simulink model "eCS_Algo_Simulation"  (R2018a)
settings: Solver=ode1  StartTime=0.0  StopTime=0.2  FixedStep=1/80000  RelTol=1e-3  EnableMultiTasking=on
PostLoadFcn:
  | , if any(exist('dsrtsu_mdlpostloadfcn', 'file') == [2, 3, 6]), try dsrtsu_mdlpostloadfcn('Execute', bdroot); catch fprintf('Error in PostLoadFcn (dsrtsu_mdlpostloadfcn) for model "%s":\n %s\n', bdroot, lasterr); end, end,
values from neighbouring files (symbols this model uses):
  AccSensor = 5    [Parameter_eCS_Algo.m]
  AlgoType = 0    [Parameter_eCS_Algo.m]
  Cxy = 1*0.017    (= 0.017)    [Acc_Init_SelV1.m]
  Cxz = 1*0.017    (= 0.017)    [Acc_Init_SelV1.m]
  Cyx = 1*0.017    (= 0.017)    [Acc_Init_SelV1.m]
  Cyz = 1*0.017    (= 0.017)    [Acc_Init_SelV1.m]
  Czx = 1*0.017    (= 0.017)    [Acc_Init_SelV1.m]
  Czy = 1*0.017    (= 0.017)    [Acc_Init_SelV1.m]
  FreqTemperature = 10    [Acc_Init_SelV1.m]
  MaxSensorOffset = 0.3    [Acc_Init_SelV1.m]
  Mean_x_noise = 4e-3    (= 0.004)    [Acc_Init_SelV1.m]
  Mean_y_noise = 4e-3    (= 0.004)    [Acc_Init_SelV1.m]
  Mean_z_noise = 4e-3    (= 0.004)    [Acc_Init_SelV1.m]
  ODR = 8000    [Acc_Init_SelV1.m]
  offsetcorrection_on_off = 0    [Parameter_eCS_Algo.m]
  pulsetype = 2    [Parameter_eCS_Algo.m]    (also in run_simulation.m = j; run_simulation_ActiveX.m = j)
  Range = 4    [Acc_Init_SelV1.m]
  TempBias = 0    [Acc_Init_SelV1.m]
  TemperatureAmp = 0    [Acc_Init_SelV1.m]
  Var_x_noise = 1.84e-9    (= 1.84e-09)    [Acc_Init_SelV1.m]
  Var_y_noise = 2.025e-09    [Acc_Init_SelV1.m]
  Var_z_noise = 1.374e-09    [Acc_Init_SelV1.m]
  w_x = 2*pi*F_x    (= 376.991118431)    [Acc_Init_SelV1.m]
  w_y = 2*pi*F_y    (= 376.991118431)    [Acc_Init_SelV1.m]
  w_z = 2*pi*F_z    (= 376.991118431)    [Acc_Init_SelV1.m]
  x_max_temp_drift = 0.061    [Acc_Init_SelV1.m]
  x_offset_enable = 0    [Acc_Init_SelV1.m]
  x_run_to_run_drift = 0.0    (= 0)    [Acc_Init_SelV1.m]
  x_temp_co_drift = 0.000    (= 0)    [Acc_Init_SelV1.m]
  Xi_x = 0.7    [Acc_Init_SelV1.m]
  Xi_y = 0.7    [Acc_Init_SelV1.m]
  Xi_z = 0.7    [Acc_Init_SelV1.m]
  y_max_temp_drift = 0.061    [Acc_Init_SelV1.m]
  y_offset_enable = 0    [Acc_Init_SelV1.m]
  y_run_to_run_drift = 0.0    (= 0)    [Acc_Init_SelV1.m]
  y_temp_co_drift = 0.000    (= 0)    [Acc_Init_SelV1.m]
  z_max_temp_drift = 0.13    [Acc_Init_SelV1.m]
  z_offset_enable = 0    [Acc_Init_SelV1.m]
  z_run_to_run_drift = 0.0    (= 0)    [Acc_Init_SelV1.m]
  z_temp_co_drift = 0.000    (= 0)    [Acc_Init_SelV1.m]
undefined symbols (not defined in the file or in its folder): controller_sample_rate, DiscIntNeverNeededParam, gmw_roada_x__m_s__, gmw_roada_y__m_s__, gmw_roadtime_2kHz, Meldorf_HindenburgstraAcceleration_x__m_s_2_, Meldorf_HindenburgstraAcceleration_y__m_s_2_, Meldorf_HindenburgstraTime__s_, pulse_FF27, pulse_MPDB, pulse_ODB40, pulse_ODB64, pulse_USNCAP, pulsetime_FF27, pulsetime_MPDB, pulsetime_ODB40, pulsetime_ODB64, pulsetime_USNCAP, sigbuilder_block, VW_416_2kHza_x_2kHz, VW_416_2kHza_y_2kHz, VW_416_2kHztime_2kHz
libraries: simulink x23, dspsigops x1
(part 1 of 2)
settings Model: DSRTSU_INTERNAL_RTI_VER=520  DSRTSU_INTERNAL_RTI_TYPE=rti1103  DSRTSU_INTERNAL_RTIFPGA=110  RTICANMMDATA=struct('GeneralSetupData',struct('modelroot','P:\ES\USER\Hinrichs\Projekte\93D48_eCS\Simulink','generalsettings',struct('filesettings',struct('destfolder',struct('Name','RTICANMM_FILES','Check',1),'buildfolder',struct('Name','.','Check',1),'AbsDestfolder',struct('Name','P:\ES\USER\Hinrichs\Projekte\93D48_eCS\Simulink\RTICANMM_FILES'),'AbsBuildfolder',struct('Name','P:\ES\USER\Hinrichs\Projekte\93D48_eCS\Simulink'))),'options',struct('addpaths',1,'rmpaths',1,'addtrcexclusion',logical(1),'cannavigator',struct('checkmonitoring',0),'show_usrtrc',0,'use_usrtrc',0),'advanced',struct('options',[1 1 1 1 1 1 1 1 1 1 1 1 1 1 1 1 1 1 1 1 1 1 1 1 1 1 1 1 1 1 1 1 1 1 1 1 1 1 1 1 1 1 1 1 1 1 1 1 1 1 1 1 1 1 1 1 1 1 1 1 1 1 1 1 1 1 1 1 1 1 1 1 1 1 1 1 1 1 1 1 1 1 1 1 1 1 1 1 1 1 1 1 1 1 1 1 1 1 1 1]),'MPSetup',{{}},'modelname','eCS_Algo_Simulation','block','eCS_Algo_Simulation'))  DSRTSU_INTERNAL_RTIFLEXRAYCONFIG=110  Creator=heiko.hinrichs  LastModifiedBy=Heiko.Hinrichs
settings SolverCC: AutoInsertRateTranBlk=on
settings DataIOCC: LimitDataPoints=on  SaveFormat=Array  SignalLoggingSaveFormat=ModelDataLogs
settings OptimizationCC: BlockReduction=off  OptimizeBlockIOStorage=off  BufferReuse=off  GlobalBufferReuse=off  ExpressionFolding=off  ExpressionDepthLimit=2147483647  LocalBlockOutputs=off  LifeSpan=inf  OptimizeDataStoreBuffers=off  BusAssignmentInplaceUpdate=off
settings DebuggingCC: UnderspecifiedInitializationDetection=Classic  MergeDetectMultiDrivingBlocksExec=none  SolverPrmCheckMsg=warning  FcnCallInpInsideContextMsg=warning  StateNameClashWarn=warning  SFUnexpectedBacktrackingDiag=warning  SFNoUnconditionalDefaultTransitionDiag=warning  SFExecutionAtInitializationDiag=none
settings HardwareCC: ProdBitPerPointer=32  ProdBitPerSizeT=32  ProdBitPerPtrDiffT=32  ProdLargestAtomicInteger=Integer  ProdEndianess=BigEndian  ProdWordSize=32  ProdHWDeviceType=Custom Processor->Custom  TargetHWDeviceType=Custom Processor->Custom
settings ModelReferenceCC: PropagateSignalLabelsOutOfModel=off
settings SFSimCC: MATLABDynamicMemAlloc=off
settings RTWCC: SystemTargetFile=rti1103.tlc  MakeCommand=make_rti  TemplateMakefile=rti1103.tmf  Description=dSPACE DS1103 Hardware Platform
settings CodeAppCC: StateflowObjectComments=on
settings STFCustomTargetCC: ParMdlRefBuildCompliant=on  GRTInterface=off  SystemTargetFile=rti1103.tlc
settings GRTTargetCC: TargetLangStandard=C89/C90 (ANSI)  CompOptLevelCompliant=off  ConcurrentExecutionCompliant=off  CombineOutputUpdateFcns=off  MatFileLogging=off  CPPClassGenCompliant=off  UseToolchainInfoCompliant=off  ExtModeMexFile=noextcomm
settings ConfigComp: CovMetricSettings=dw  CovHtmlReporting=on  CovSaveCumulativeToWorkspaceVar=on  CovSaveSingleToWorkspaceVar=on  CovExternalEMLEnable=off

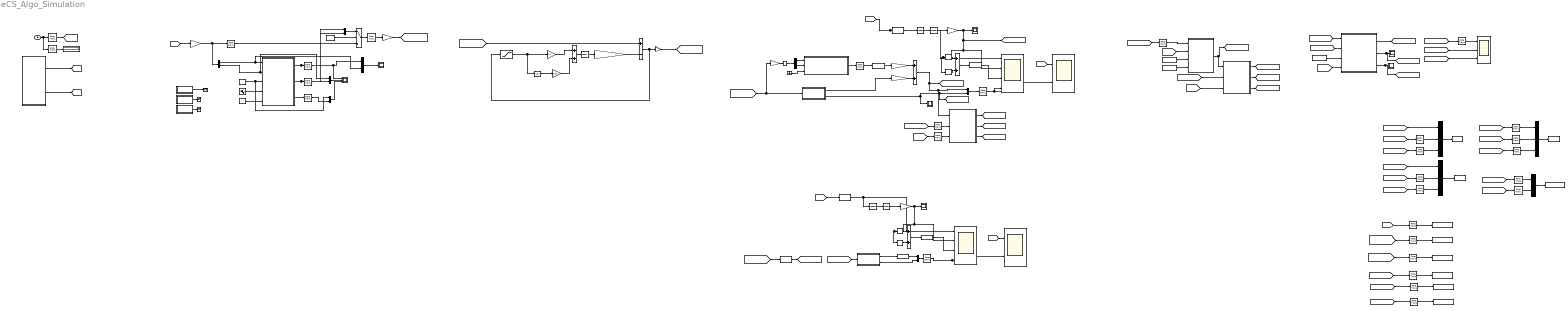
== system eCS_Algo_Simulation ==
  note: "retractor locked"
  note: Outputs
  note: Retractor mechanics
  note: Solenoid
  note: eCS algo
  note: Offset correction
  note: Input pulses / load cases
  note: "old" algo unidirectional
  note: Sensor model Ziad
  note: "lever locked" (solenoid locked)
  note: "lock decision" (algo "locked")
  Accelerometer : Subsystem
  Add{,1,3..4} (4 alike) : Sum
  Add2 : Sum  Inputs=+-
  Clock : Clock
  Compare To Constant : simulink/Logic and Bit Operations/Compare To Constant  relop=>=  const=25  OutDataTypeStr=uint8
  Compare To Constant1 : simulink/Logic and Bit Operations/Compare To Constant  relop=>=  const=50  OutDataTypeStr=uint8
  Compare To Constant2 : simulink/Logic and Bit Operations/Compare To Constant  relop=>=  const=25  OutDataTypeStr=uint8
  Compare To Constant3 : simulink/Logic and Bit Operations/Compare To Constant  relop=>=  const=50  OutDataTypeStr=uint8
  Constant : Constant  Value=0
  Crash signal1 : Subsystem  Tag=STV Subsys  LoadFcn=sigbuilder_block('load');  StartFcn=sigbuilder_block('start');  StopFcn=sigbuilder_block('stop');  ClipboardFcn=sigbuilder_block('clipboard');  mask(Sigbuilder block){tuvar=[0:10]}
      mask help: Simulink:masks:SigbuilderBlock_MD
      mask init:
      | if ~strcmp(get_param(bdroot(gcbh),'SimulationStatus'),'stopped') tuvar = sigbuilder_block('maskInit'); end
      settings: CopyFcn=sigbuilder_block('copy');  DeleteFcn=sigbuilder_block('delete');  ModelCloseFcn=sigbuilder_block('modelClose');  PreSaveFcn=sigbuilder_block('preSave');  PauseFcn=sigbuilder_block('pause');  ContinueFcn=sigbuilder_block('continue');  NameChangeFcn=sigbuilder_block('namechange');  OpenFcn=sigbuilder_block('open',[50.25 1.5 1200 576 ]);  CloseFcn=sigbuilder_block('close');
      mask Display: plot(0, 0, 100, 100,[2, 2, 32, 32, 2], [68, 8, 8, 68, 68],[32, 2], [38, 38], [32, 19, 2],[53, 60, 44], [32, 17, 17, 2],[16, 16, 31, 31]);txt = getActiveGroup(gcbh);text(2, 100, txt,'verticalAlignment', 'top');
  Crash signal3 : Subsystem  Tag=STV Subsys  LoadFcn=sigbuilder_block('load');  StartFcn=sigbuilder_block('start');  StopFcn=sigbuilder_block('stop');  ClipboardFcn=sigbuilder_block('clipboard');  mask(Sigbuilder block){tuvar=[0:10]}
      mask help: Simulink:masks:SigbuilderBlock_MD
      mask init:
      | if ~strcmp(get_param(bdroot(gcbh),'SimulationStatus'),'stopped') tuvar = sigbuilder_block('maskInit'); end
      settings: CopyFcn=sigbuilder_block('copy');  DeleteFcn=sigbuilder_block('delete');  ModelCloseFcn=sigbuilder_block('modelClose');  PreSaveFcn=sigbuilder_block('preSave');  PauseFcn=sigbuilder_block('pause');  ContinueFcn=sigbuilder_block('continue');  NameChangeFcn=sigbuilder_block('namechange');  OpenFcn=sigbuilder_block('open',[54 1.5 1200 540 ]);  CloseFcn=sigbuilder_block('close');
      mask Display: plot(0, 0, 100, 100,[2, 2, 32, 32, 2], [68, 8, 8, 68, 68],[32, 2], [38, 38], [32, 19, 2],[53, 60, 44], [32, 17, 17, 2],[16, 16, 31, 31]);txt = getActiveGroup(gcbh);text(2, 100, txt,'verticalAlignment', 'top');
  Demux : Demux  Outputs=2
  Demux2 : Demux  Outputs=2
  Discrete-Time Integrator{,1..3} (4 alike) : DiscreteIntegrator  SampleTime=-1  ICPrevOutput=DiscIntNeverNeededParam  ICPrevScaledInput=DiscIntNeverNeededParam
  Discrete-Time Integrator4 : DiscreteIntegrator  gainval=1  SampleTime=-1  LimitOutput=on  UpperSaturationLimit=0.3 * 9.81  LowerSaturationLimit=-0.3 * 9.81  ICPrevOutput=DiscIntNeverNeededParam  ICPrevScaledInput=DiscIntNeverNeededParam
  G-lock Scope : Scope  NumInputPorts=4
  G-lock Scope new : Scope  NumInputPorts=4
  Gain : Gain  Gain=AlgoType
  Gain1 : Gain  Gain=1- AlgoType
  Ground : Ground
  Input (Pulse/ Angle) : Subsystem
  Mux : Mux  Inputs=3
  Mux{1,3,5..9} (7 alike) : Mux  Inputs=2
  Mux2 : Mux  Inputs=3
  Mux4 : Mux  Inputs=3
  Noisy : Subsystem  Tag=STV Subsys  LoadFcn=sigbuilder_block('load');  StartFcn=sigbuilder_block('start');  StopFcn=sigbuilder_block('stop');  ClipboardFcn=sigbuilder_block('clipboard');  mask(Sigbuilder block){tuvar=[0:10]}
      mask help: Simulink:masks:SigbuilderBlock_MD
      mask init:
      | if ~strcmp(get_param(bdroot(gcbh),'SimulationStatus'),'stopped') tuvar = sigbuilder_block('maskInit'); end
      settings: CopyFcn=sigbuilder_block('copy');  DeleteFcn=sigbuilder_block('delete');  ModelCloseFcn=sigbuilder_block('modelClose');  PreSaveFcn=sigbuilder_block('preSave');  PauseFcn=sigbuilder_block('pause');  ContinueFcn=sigbuilder_block('continue');  NameChangeFcn=sigbuilder_block('namechange');  OpenFcn=sigbuilder_block('open',[54 1.5 1200 535.5 ]);  CloseFcn=sigbuilder_block('close');
      mask Display: plot(0, 0, 100, 100,[2, 2, 32, 32, 2], [68, 8, 8, 68, 68],[32, 2], [38, 38], [32, 19, 2],[53, 60, 44], [32, 17, 17, 2],[16, 16, 31, 31]);txt = getActiveGroup(gcbh);text(2, 100, txt,'verticalAlignment', 'top');
  Output Scope : Scope  NumInputPorts=3
  Pulse measured : RateTransition
  Pulse measured1 : RateTransition  Deterministic=off  OutPortSampleTime=1/2000
  Pulse measured2 : RateTransition
  Pulse raw (g) : Gain  Gain=1/9.807
  Pulse raw / measured by sensor : Scope
  Pulse raw1 : Gain  Gain=9.807
  Pulse with Offsetcorr. : Gain
  RT : RateTransition  OutPortSampleTime=0.0001
  Rate Transition{,1..11,15,22} (14 alike) : RateTransition
  Rate Transition{12..14,16..21,23..24} (11 alike) : RateTransition  OutPortSampleTime=1/10000
  Rate Transition25 : RateTransition  OutPortSampleTime=1/5
  "Saturation acc. script, i.e.+-0,3g (max. offset of sensor after ageing)" : Saturate  UpperLimit=MaxSensorOffset * 9.807  LowerLimit=-MaxSensorOffset * 9.807
  Scope : Scope
  Scope1 : Scope  NumInputPorts=3
  Sign : Signum
  Temperature : Sin  Amplitude=TemperatureAmp  Bias=TempBias  Frequency=FreqTemperature  SampleTime=0
  Terminator : Terminator
  Terminator2 : Terminator
  Terminator3 : Terminator
  Tilt_Lock_Scop : Scope  NumInputPorts=2
  Tilt_Lock_Scop1 : Scope  NumInputPorts=2
  To Workspace : ToWorkspace  VariableName=triggers_s  SaveFormat=Timeseries  SampleTime=-1
      settings: MaxDataPoints=1  Save2DSignal=2-D array (concatenate along first dimension)
  To Workspace1 : ToWorkspace  VariableName=pulse  SaveFormat=Timeseries  SampleTime=-1
      settings: Save2DSignal=2-D array (concatenate along first dimension)
  To Workspace2 : ToWorkspace  VariableName=pulse_sensor_output  SaveFormat=Timeseries  SampleTime=-1
      settings: Save2DSignal=2-D array (concatenate along first dimension)
  To Workspace3 : ToWorkspace  VariableName=pulse_with_offsetcorrection  SaveFormat=Timeseries  SampleTime=-1
      settings: Save2DSignal=2-D array (concatenate along first dimension)
  To Workspace4 : ToWorkspace  VariableName=s_ball  SaveFormat=Timeseries  SampleTime=-1
      settings: Save2DSignal=2-D array (concatenate along first dimension)
  To Workspace5 : ToWorkspace  VariableName=trigger_eCS  SaveFormat=Timeseries  SampleTime=-1
      settings: Save2DSignal=2-D array (concatenate along first dimension)
  To Workspace6 : ToWorkspace  VariableName=triggers_times  SaveFormat=Timeseries  SampleTime=-1
      settings: MaxDataPoints=1  Save2DSignal=2-D array (concatenate along first dimension)
  To Workspace7 : ToWorkspace  VariableName=s_rig  SaveFormat=Timeseries  SampleTime=-1
      settings: Save2DSignal=2-D array (concatenate along first dimension)
  To Workspace8 : ToWorkspace  VariableName=s_locking  SaveFormat=Timeseries  SampleTime=-1
      settings: Save2DSignal=2-D array (concatenate along first dimension)
  To Workspace9 : ToWorkspace  VariableName=triggercounts  SaveFormat=Timeseries  SampleTime=-1
      settings: Save2DSignal=2-D array (concatenate along first dimension)
  Vektor_addition_Pulse : Fcn  Expr=sqrt( (u(1)*u(1)) + (u(2)*u(2)) )
  Vektor_addition_Pulse1 : Fcn  Expr=sqrt( (u(1)*u(1)) + (u(2)*u(2)) )
  Vektor_addition_Pulse2 : Fcn  Expr=sqrt( (u(1)*u(1)) + (u(2)*u(2)) )
  acc. measurement direct/via acc. sensor : Switch  Criteria=u2 > Threshold
  "acc. sensor type: 0=direct, 1=AD, 2=ST, 3=TDK, 4=NXP" : Constant  Value=AccSensor  VectorParams1D=off
  delta-t to lock (ms) : Constant  Value=5
  delta-t to unlock (ms) : Constant  Value=7
  deviation dependent correction: 0.1/s ~10mg/s at 1m/s²deviation ~0,6°/s with saturation +-0,3g: max. 30mg/s / ~1,8°/s possible : Gain  Gain=0.1
  eCS Algo : Subsystem
  eCS Algo new : Subsystem
  locking distance (mm) : Constant  Value=18.13
  m/s² to g : Gain  Gain=1/9.807
  offset correction on/off : Gain  Gain=offsetcorrection_on_off  OutMin=[0]  OutMax=[1]
  permanent correction: 0.01m/s²/s ~1mg/s ~0,06°/s : Gain  Gain=0.01
  retractor locking trigger : MATLAB Function  TreatAsAtomicUnit=on
  s-locking retractor (mm) : Scope
  s-rig (mm) : Scope
  s-rig (mm) new : Scope
  s-rig-trigger : DataTypeConversion
  s-rig-trigger new : DataTypeConversion
  s-rig-trigger new1 : DataTypeConversion
  s_rig in mm : Gain  Gain=1000
  s_rig in mm1 : Gain  Gain=1000
  solenoid time delay : MATLAB Function  TreatAsAtomicUnit=on
  time (0.2s-steps) : Display
  "trigger travels, times and counts" : MATLAB Function  TreatAsAtomicUnit=on
  "trigger travels, times and counts1" : MATLAB Function  TreatAsAtomicUnit=on
  trigger_lock : DataTypeConversion
  triggertime_retractor (ms) : Scope
  zero 1 : Constant  Value=0
  µC Signalverarbeitung und Algorithmus2 : Subsystem
  wires:
  Mux1/1 -> Rate Transition3/1
  eCS Algo/1(Trigger eCS) -> trigger_lock/1
  Discrete-Time Integrator1/1 -> s_rig in mm/1
  Input (Pulse/ Angle)/1("Pulse_profile ") -> [Pulse]  "pulse in m/s²"
  Discrete-Time Integrator/1 -> Discrete-Time Integrator1/1
  eCS Algo new/2(s_ball) -> [s_ball], Mux3/2, Scope/1
  Add4/1 -> "trigger travels, times and counts"/1(trigger), Mux3/1, [trigger_eCS]
  trigger_lock/1 -> Mux1/1
  eCS Algo/2(s_ball) -> Mux1/2
  s_rig in mm/1 -> [s], G-lock Scope new/2, Compare To Constant/1, Compare To Constant1/1, s-rig (mm) new/1
  [angle] -> Tilt_Lock_Scop/1
  Input (Pulse/ Angle)/2(angle in °) -> [angle]
  Vektor_addition_Pulse/1 -> [Pulse_unidirectional]
  [Pulse_unidirectional] -> eCS Algo/1(Pulse)
  Discrete-Time Integrator2/1 -> Discrete-Time Integrator3/1
  Discrete-Time Integrator3/1 -> s_rig in mm1/1
  Vektor_addition_Pulse2/1 -> Discrete-Time Integrator2/1, G-lock Scope/1
  Compare To Constant/1 -> Add/2
  Compare To Constant1/1 -> Add/1
  Compare To Constant2/1 -> Add1/2
  Compare To Constant3/1 -> Add1/1
  s_rig in mm1/1 -> G-lock Scope/2, Compare To Constant2/1, Compare To Constant3/1, s-rig (mm)/1
  Add1/1 -> s-rig-trigger/1
  s-rig-trigger/1 -> G-lock Scope/3
  Add/1 -> s-rig-trigger new/1
  Mux3/1 -> Rate Transition4/1
  s-rig-trigger new/1 -> G-lock Scope new/3
  "Saturation acc. script, i.e.+-0,3g (max. offset of sensor after ageing)"/1 -> Sign/1, deviation dependent correction: 0.1/s ~10mg/s at 1m/s²deviation ~0,6°/s with saturation +-0,3g: max. 30mg/s / ~1,8°/s possible/1
  Sign/1 -> permanent correction: 0.01m/s²/s ~1mg/s ~0,06°/s/1
  offset correction on/off/1 -> Add2/2
  Discrete-Time Integrator4/1 -> offset correction on/off/1
  Add3/1 -> Discrete-Time Integrator4/1
  deviation dependent correction: 0.1/s ~10mg/s at 1m/s²deviation ~0,6°/s with saturation +-0,3g: max. 30mg/s / ~1,8°/s possible/1 -> Add3/1
  permanent correction: 0.01m/s²/s ~1mg/s ~0,06°/s/1 -> Add3/2
  Add2/1 -> Pulse with Offsetcorr./1, "Saturation acc. script, i.e.+-0,3g (max. offset of sensor after ageing)"/1
  [angle] -> Tilt_Lock_Scop1/1
  Clock/1 -> Rate Transition25/1, Rate Transition2/1
  [time] -> solenoid time delay/2(time)
  [trigger_eCS] -> Rate Transition/1
  solenoid time delay/1(trigger_out) -> "trigger travels, times and counts1"/1(trigger), [locking_solenoid]
  [locking_solenoid] -> Scope1/2
  [trigger_eCS] -> Rate Transition1/1
  Temperature/1 -> Accelerometer/4(Temperature)
  Pulse measured/1 -> Output Scope/1, Mux5/1
  Rate Transition7/1 -> Mux6/2
  Constant/1 -> Accelerometer/5(Max temp. drift)
  Accelerometer/2(Out Y) -> Mux8/2, Rate Transition7/1
  Accelerometer/1(Out X) -> Mux8/1, Pulse measured/1
  Mux7/1 -> Output Scope/3
  Demux2/2 -> Accelerometer/2(In Y), Mux6/1
  Accelerometer/3(Out Z) -> Rate Transition8/1
  zero 1/1 -> Accelerometer/3(In Z), Mux7/1
  Mux6/1 -> Output Scope/2
  Mux5/1 -> Pulse raw / measured by sensor/1
  Crash signal1/1(Signal 1) -> Terminator/1
  Demux2/1 -> Mux5/2, Accelerometer/1(In X)
  Rate Transition8/1 -> Mux7/2
  Pulse with Offsetcorr./1 -> [Pulse_with_offsetcorrection]
  locking distance (mm)/1 -> retractor locking trigger/3(s_mech_locking)
  [time] -> retractor locking trigger/4(time)
  [s] -> retractor locking trigger/2(s)
  [locking_solenoid] -> retractor locking trigger/1(trigger_solenoid)
  [locking_retractor] -> Scope1/3
  retractor locking trigger/1(trigger_retractor) -> [locking_retractor]
  retractor locking trigger/2(triggertime_retractor) -> [triggertime_retractor], triggertime_retractor (ms)/1
  retractor locking trigger/3(s_locking) -> [s_locking_retractor], s-locking retractor (mm)/1
  Pulse measured1/1 -> Pulse raw1/1
  Pulse raw1/1 -> [Pulse_no_offsetcorrection]
  [Pulse_with_offsetcorrection] -> Vektor_addition_Pulse/1
  [Pulse] -> Vektor_addition_Pulse1/1, G-lock Scope new/1
  [Pulse] -> Vektor_addition_Pulse2/1
  Vektor_addition_Pulse1/1 -> Discrete-Time Integrator/1
  [Pulse_no_offsetcorrection] -> Add2/1
  Noisy/1(Signal 1) -> Terminator2/1
  Crash signal3/1(Signal 1) -> Terminator3/1
  Rate Transition/1 -> solenoid time delay/1(trigger)
  Rate Transition1/1 -> Scope1/1
  Mux/1 -> To Workspace/1
  Pulse raw (g)/1 -> Pulse measured2/1, Demux2/1
  Rate Transition2/1 -> [time]
  [Pulse] -> Pulse raw (g)/1
  Rate Transition3/1 -> G-lock Scope/4, Tilt_Lock_Scop/2
  Rate Transition4/1 -> G-lock Scope new/4, Tilt_Lock_Scop1/2
  [time] -> Rate Transition5/1
  Rate Transition5/1 -> "trigger travels, times and counts"/3(time)
  "trigger travels, times and counts"/2(triggertime) -> [triggertime_eCS]
  [s_locking_retractor] -> Rate Transition6/1
  Rate Transition6/1 -> Mux/3
  [triggertime_eCS] -> Mux2/1
  [triggertime_solenoid] -> Rate Transition9/1
  Rate Transition9/1 -> Mux2/2
  [triggertime_retractor] -> Rate Transition10/1
  Rate Transition10/1 -> Mux2/3
  "trigger travels, times and counts"/1(s_locking) -> [s_locking_eCS]
  [s] -> Rate Transition11/1
  Rate Transition11/1 -> "trigger travels, times and counts"/2(s)
  [s_locking_eCS] -> Mux/1
  [s] -> "trigger travels, times and counts1"/2(s)
  [time] -> "trigger travels, times and counts1"/3(time)
  "trigger travels, times and counts1"/2(triggertime) -> [triggertime_solenoid]
  "trigger travels, times and counts1"/1(s_locking) -> [s_locking_solenoid]
  [s_locking_solenoid] -> Rate Transition15/1
  Rate Transition15/1 -> Mux/2
  delta-t to unlock (ms)/1 -> solenoid time delay/4(dt_to_unlock)
  delta-t to lock (ms)/1 -> solenoid time delay/3(dt_to_lock)
  acc. measurement direct/via acc. sensor/1 -> Pulse measured1/1
  Mux8/1 -> acc. measurement direct/via acc. sensor/1
  "acc. sensor type: 0=direct, 1=AD, 2=ST, 3=TDK, 4=NXP"/1 -> acc. measurement direct/via acc. sensor/2
  Pulse measured2/1 -> acc. measurement direct/via acc. sensor/3
  [Pulse] -> Rate Transition16/1
  Rate Transition16/1 -> To Workspace1/1
  Rate Transition17/1 -> To Workspace2/1
  [Pulse_no_offsetcorrection] -> Rate Transition17/1
  Rate Transition18/1 -> To Workspace3/1
  [Pulse_with_offsetcorrection] -> Rate Transition18/1
  Rate Transition19/1 -> To Workspace4/1
  [s_ball] -> Rate Transition19/1
  [trigger_eCS] -> Rate Transition20/1
  Rate Transition20/1 -> To Workspace5/1
  Mux2/1 -> To Workspace6/1
  Rate Transition13/1 -> To Workspace7/1
  [s] -> Rate Transition13/1
  Rate Transition12/1 -> Mux4/2
  [s_locking_solenoid] -> Rate Transition12/1
  [s_locking_eCS] -> Rate Transition21/1
  Rate Transition14/1 -> Mux4/3
  [s_locking_retractor] -> Rate Transition14/1
  Mux4/1 -> To Workspace8/1
  Rate Transition21/1 -> Mux4/1
  [Pulse_with_offsetcorrection] -> m/s² to g/1, eCS Algo new/1(Pulse)
  Ground/1 -> µC Signalverarbeitung und Algorithmus2/3(Acceleration z-Axis (g))
  Demux/1 -> µC Signalverarbeitung und Algorithmus2/1(Acceleration x-Axis (g))
  Demux/2 -> µC Signalverarbeitung und Algorithmus2/2(Acceleration y-Axis (g))
  Rate Transition22/1 -> s-rig-trigger new1/1
  RT/1 -> Demux/1
  eCS Algo new/1(Trigger eCS) -> Gain1/1
  µC Signalverarbeitung und Algorithmus2/1(no lock / lock [bool]) -> Rate Transition22/1
  m/s² to g/1 -> RT/1
  s-rig-trigger new1/1 -> Gain/1
  Gain/1 -> Add4/1
  Gain1/1 -> Add4/2
  "trigger travels, times and counts"/3(triggercounts) -> [triggercounts_eCS]
  "trigger travels, times and counts1"/3(triggercounts) -> [triggercounts_solenoid]
  Mux9/1 -> To Workspace9/1
  [triggercounts_solenoid] -> Rate Transition24/1
  [triggercounts_eCS] -> Rate Transition23/1
  Rate Transition23/1 -> Mux9/1
  Rate Transition24/1 -> Mux9/2
  Rate Transition25/1 -> time (0.2s-steps)/1

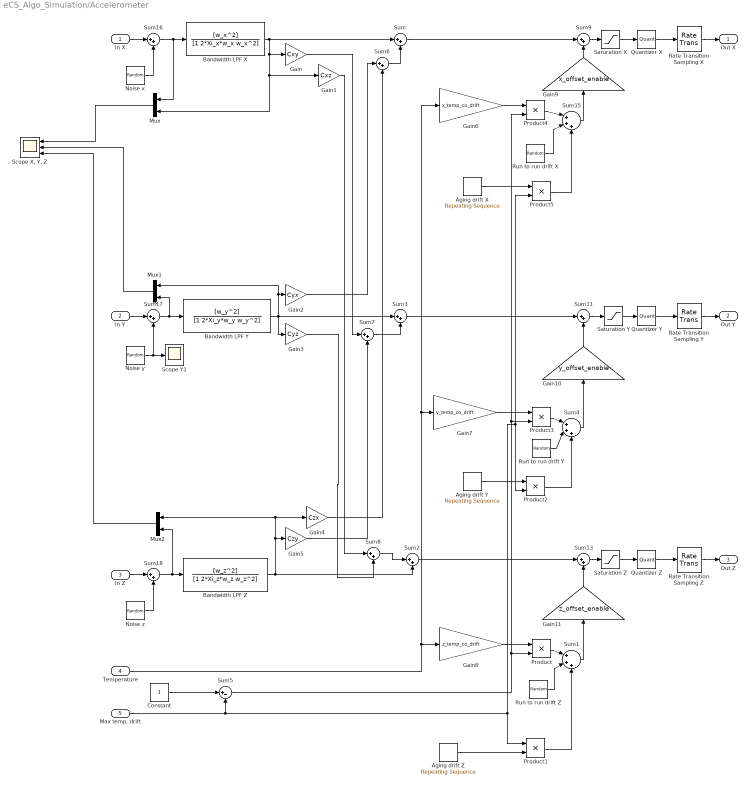
== system eCS_Algo_Simulation/Accelerometer ==
  In X : Inport
  In Y : Inport  Port=2
  In Z : Inport  Port=3
  Temperature : Inport  Port=4
  Max temp. drift : Inport  Port=5
  Aging drift X : simulink/Sources/Repeating Sequence  rep_seq_t=[0 0.1]  rep_seq_y=[0 x_max_temp_drift]
  Aging drift Y : simulink/Sources/Repeating Sequence  rep_seq_t=[0 1000]  rep_seq_y=[0 y_max_temp_drift]
  Aging drift Z : simulink/Sources/Repeating Sequence  rep_seq_t=[0 0.001]  rep_seq_y=[0 z_max_temp_drift]
  Bandwidth LPF X : TransferFcn  Numerator=[w_x^2]  Denominator=[1 2*Xi_x*w_x w_x^2]
  Bandwidth LPF Y : TransferFcn  Numerator=[w_y^2]  Denominator=[1 2*Xi_y*w_y w_y^2]
  Bandwidth LPF Z : TransferFcn  Numerator=[w_z^2]  Denominator=[1 2*Xi_z*w_z w_z^2]
  Constant : Constant
  Gain : Gain  Gain=Cxy
  Gain1 : Gain  Gain=Cxz
  Gain10 : Gain  Gain=y_offset_enable
  Gain11 : Gain  Gain=z_offset_enable
  Gain2 : Gain  Gain=Cyx
  Gain3 : Gain  Gain=Cyz
  Gain4 : Gain  Gain=Czx
  Gain5 : Gain  Gain=Czy
  Gain6 : Gain  Gain=x_temp_co_drift
  Gain7 : Gain  Gain=y_temp_co_drift
  Gain8 : Gain  Gain=z_temp_co_drift
  Gain9 : Gain  Gain=x_offset_enable
  Mux : Mux  Inputs=2
  Mux1 : Mux  Inputs=2
  Mux2 : Mux  Inputs=2
  Noise x : RandomNumber  Mean=Mean_x_noise  Variance=Var_x_noise
  Noise y : RandomNumber  Mean=Mean_y_noise  Variance=Var_y_noise
  Noise z : RandomNumber  Mean=Mean_z_noise  Variance=Var_z_noise
  Product{,1..5} (6 alike) : Product  RndMeth=Zero
  Quantizer X : Quantizer  QuantizationInterval=Resolution
  Quantizer Y : Quantizer  QuantizationInterval=Resolution
  Quantizer Z : Quantizer  QuantizationInterval=Resolution
  Rate Transition Sampling X : RateTransition  OutPortSampleTime=1/ODR
  Rate Transition Sampling Y : RateTransition  OutPortSampleTime=1/ODR
  Rate Transition Sampling Z : RateTransition  OutPortSampleTime=1/ODR
  Run to run drift X : RandomNumber  Mean=x_run_to_run_drift  Variance=0.00001
  Run to run drift Y : RandomNumber  Mean=y_run_to_run_drift  Variance=0.00001
  Run to run drift Z : RandomNumber  Mean=z_run_to_run_drift  Variance=0.00001
  Saturation X : Saturate  UpperLimit=Range  LowerLimit=-Range
  Saturation Y : Saturate  UpperLimit=Range  LowerLimit=-Range
  Saturation Z : Saturate  UpperLimit=Range  LowerLimit=-Range
  "Scope X, Y, Z" : Scope  NumInputPorts=3
  Scope Y1 : Scope
  Sum{,2..3,6..9,11,13,16..18} (12 alike) : Sum  Inputs=|++
  Sum1 : Sum  Inputs=|+++
  Sum15 : Sum  Inputs=|+++
  Sum4 : Sum  Inputs=|+++
  Sum5 : Sum  Inputs=|+-
  Out X : Outport
  Out Y : Outport  Port=2
  Out Z : Outport  Port=3
  wires:
  Run to run drift Z/1 -> Sum1/2
  Sum4/1 -> Gain10/1
  Run to run drift Y/1 -> Sum4/2
  Sum1/1 -> Gain11/1
  Bandwidth LPF Y/1 -> Gain3/1, Sum3/1, Mux1/1, Gain2/1
  Sum6/1 -> Sum/2
  Gain4/1 -> Sum6/2
  Bandwidth LPF Z/1 -> Mux2/1, Gain4/1, Gain5/1, Sum2/2
  Quantizer X/1 -> Rate Transition Sampling X/1
  Saturation Y/1 -> Quantizer Y/1
  Quantizer Z/1 -> Rate Transition Sampling Z/1
  Sum7/1 -> Sum3/2
  Gain5/1 -> Sum7/2
  Saturation X/1 -> Quantizer X/1
  Sum/1 -> Sum9/1
  Sum9/1 -> Saturation X/1
  Gain2/1 -> Sum6/1
  Sum3/1 -> Sum11/1
  Sum2/1 -> Sum13/1
  Sum13/1 -> Saturation Z/1
  Gain1/1 -> Sum8/1
  Run to run drift X/1 -> Sum15/2
  Gain3/1 -> Sum8/2
  Sum15/1 -> Gain9/1
  Sum11/1 -> Saturation Y/1
  In X/1 -> Sum16/1
  Sum16/1 -> Mux/1, Bandwidth LPF X/1
  Bandwidth LPF X/1 -> Mux/2, Gain1/1, Gain/1, Sum/1
  Gain/1 -> Sum7/1
  Quantizer Y/1 -> Rate Transition Sampling Y/1
  Saturation Z/1 -> Quantizer Z/1
  Noise z/1 -> Sum18/2
  Rate Transition Sampling Y/1 -> Out Y/1
  Sum17/1 -> Mux1/2, Bandwidth LPF Y/1
  Sum18/1 -> Bandwidth LPF Z/1, Mux2/2
  In Z/1 -> Sum18/1
  In Y/1 -> Sum17/1
  Rate Transition Sampling X/1 -> Out X/1
  Noise y/1 -> Scope Y1/1, Sum17/2
  Rate Transition Sampling Z/1 -> Out Z/1
  Noise x/1 -> Sum16/2
  Mux2/1 -> "Scope X, Y, Z"/3
  Temperature/1 -> Gain6/1, Gain7/1, Gain8/1
  Mux/1 -> "Scope X, Y, Z"/1
  Constant/1 -> Sum5/1
  Max temp. drift/1 -> Product2/2, Product5/2, Product1/1, Sum5/2
  Gain8/1 -> Product/1
  Product/1 -> Sum1/1
  Sum5/1 -> Product4/2, Product3/2, Product/2
  Product1/1 -> Sum1/3
  Aging drift Z/1 -> Product1/2
  Gain7/1 -> Product3/1
  Product3/1 -> Sum4/1
  Gain6/1 -> Product4/1
  Product4/1 -> Sum15/1
  Aging drift X/1 -> Product5/1
  Product5/1 -> Sum15/3
  Product2/1 -> Sum4/3
  Aging drift Y/1 -> Product2/1
  Sum8/1 -> Sum2/1
  Mux1/1 -> "Scope X, Y, Z"/2
  Gain9/1 -> Sum9/2
  Gain10/1 -> Sum11/2
  Gain11/1 -> Sum13/2

== system eCS_Algo_Simulation/Crash signal1 ==
  Demux : Demux  Tag=STV Demux  Outputs=1
  FromWs : FromWorkspace  Tag=STV FromWs  VariableName=tuvar  SampleTime=0
      SigBuilderData=|
      | common.afterFinalStr = 'Extrapolate'
      | common.sampleTime = 0
      | dataSet.timeRange = [0 0.01]
      | dataSet.name = 'Group 1'
      | sbobj.Groups.Name = 'Group 1'
      | sbobj.Groups.Signals.Name = 'Signal 1'
      | sbobj.Groups.Signals.XData = [0 0.0005 0.001 0.001 0.0015 0.002 0.0025 0.00299 0.00299 0.0035 0.004 0.004 0.0045 0.0045 0.005 0.005 0.0055 0.0055 0.006 0.006 0.0065 0.007 0.007 0.0075 0.008 0.008 0.0085 0.009 0.0095 0.0095 0.01]
      | sbobj.Groups.Signals.YData = [0 2 2 1.99 2 2 2 2 0 0 0.015 0.02 0.005 0 2 2.005 3.96 3.98 6.04 6.03 6.02 6.04 6.06 6 5.98 0 -0.02 6 -0.02 0 0]
      | sbobj.Groups.TimeRange = [0 0.01]
  Signal 1 : Outport  Tag=STV Outport
  wires:
  Demux/1 -> Signal 1/1
  FromWs/1 -> Demux/1

== system eCS_Algo_Simulation/Crash signal3 ==
  Demux : Demux  Tag=STV Demux  Outputs=1
  FromWs : FromWorkspace  Tag=STV FromWs  VariableName=tuvar  SampleTime=0
      SigBuilderData=|
      | common.afterFinalStr = 'Extrapolate'
      | common.sampleTime = 0
      | dataSet.timeRange = [0 0.01]
      | dataSet.name = 'Group 1'
      | sbobj.Groups.Name = 'Group 1'
      | sbobj.Groups.Signals.Name = 'Signal 1'
      | sbobj.Groups.Signals.XData = [0 0.0005 0.001 0.001 0.0015 0.002 0.0025 0.003 0.003 0.0035 0.004 0.004 0.0045 0.0045 0.005 0.005 0.0055 0.0055 0.006 0.006 0.0065 0.007 0.007 0.0075 0.008 0.008 0.0085 0.009 0.0095 0.0095 0.01]
      | sbobj.Groups.Signals.YData = [0 2 2 1.99 2 2 2 2 0 0 0.015 0.02 0.005 0 2 2.005 3.96 3.98 6.04 6.03 6.02 6.04 6.06 6 5.98 0 -0.02 6 -0.02 0 0]
      | sbobj.Groups.TimeRange = [0 0.01]
  Signal 1 : Outport  Tag=STV Outport
  wires:
  Demux/1 -> Signal 1/1
  FromWs/1 -> Demux/1

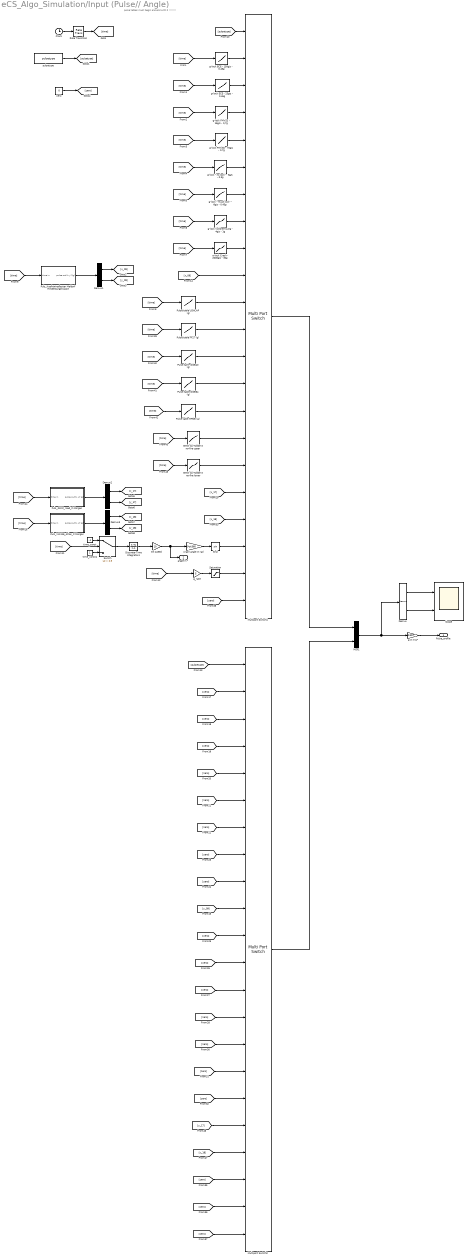
== system eCS_Algo_Simulation/Input (Pulse// Angle) ==
  note: pulse tables must begin and end with 0 !!!!!!!
  BMW QV72003-3 no-fire lower : Lookup_n-D  NumberOfTableDimensions=1  BreakpointsForDimension1=[-0.011 0.00 0.020 0.045 0.059]  Table=[0 0 11.0 11.0 0]  ExtrapMethod=Clip  UseLastTableValue=on  InternalRulePriority=Speed  RndMeth=Simplest  InputSameDT=on
  BMW QV72003-3 no-fire upper : Lookup_n-D  NumberOfTableDimensions=1  BreakpointsForDimension1=[0 0.027 0.059 0.085]  Table=[0 16.2 16.2 0]  ExtrapMethod=Clip  UseLastTableValue=on  InternalRulePriority=Speed  RndMeth=Simplest  InputSameDT=on
  Clock : Clock
  Demux{,1..3} (4 alike) : Demux  Outputs=2
  Discrete-Time Integrator4 : DiscreteIntegrator  gainval=1  SampleTime=-1  UpperSaturationLimit=0.3 * 9.81  LowerSaturationLimit=-0.3 * 9.81  ICPrevOutput=DiscIntNeverNeededParam  ICPrevScaledInput=DiscIntNeverNeededParam
  Multiport Switch1 : MultiPortSwitch  Inputs=20  DataPortForDefault=Additional data port
  Multiport Switch2 : MultiPortSwitch  Inputs=20  DataPortForDefault=Additional data port
  Mux1 : Mux  Inputs=2
  Puls_GWM_road_C.Morgan : Subsystem
  Puls_Kopfsteinpflaster Meldorf Hindenburgstrasse : Subsystem
  Puls_VW416_Atlas_C.Morgan : Subsystem
  Pulse table FF27 (g) : Lookup  InputValues=pulsetime_FF27  Table=pulse_FF27  LookUpMeth=Interpolation-Use End Values
  Pulse table MPDB (g) : Lookup  InputValues=pulsetime_MPDB  Table=pulse_MPDB  LookUpMeth=Interpolation-Use End Values
  Pulse table ODB40 (g) : Lookup  InputValues=pulsetime_ODB40  Table=pulse_ODB40  LookUpMeth=Interpolation-Use End Values
  Pulse table ODB64 (g) : Lookup  InputValues=pulsetime_ODB64  Table=pulse_ODB64  LookUpMeth=Interpolation-Use End Values
  Pulse table USNCAP (g) : Lookup  InputValues=pulsetime_USNCAP  Table=pulse_USNCAP  LookUpMeth=Interpolation-Use End Values
  Rate Transition : RateTransition
  Saturation : Saturate  UpperLimit=5  LowerLimit=0
  Scope : Scope  NumInputPorts=2
  Sin2 : Trigonometry
  Switch : Switch  Criteria=u2 > Threshold  Threshold=2.5
  crash angle in rad : Gain  Gain=2*pi/360
  g in m/s² : Gain  Gain=9.807
  "g-lock \" must lock\" - 6g/s - 0.45g" : Lookup_n-D  NumberOfTableDimensions=1  BreakpointsForDimension1=[0 0.075 0.3 0.4]  Table=[0 0.45 0.45 0]  ExtrapMethod=Clip  UseLastTableValue=on  InternalRulePriority=Speed  RndMeth=Simplest  InputSameDT=on
  "g-lock \" no lock\" - 6g/s - 0.3g" : Lookup_n-D  NumberOfTableDimensions=1  BreakpointsForDimension1=[0 0.050 0.5 0.6]  Table=[0 0.3 0.3 0]  ExtrapMethod=Clip  UseLastTableValue=on  InternalRulePriority=Speed  RndMeth=Simplest  InputSameDT=on
  g-lock Crash - 2000g/s - 30g : Lookup_n-D  NumberOfTableDimensions=1  BreakpointsForDimension1=[0 0.015 0.055 0.08]  Table=[0 30 30 0]  ExtrapMethod=Clip  UseLastTableValue=on  InternalRulePriority=Speed  RndMeth=Simplest  InputSameDT=on
  g-lock ECE - 150g/s - 0.45g : Lookup_n-D  NumberOfTableDimensions=1  BreakpointsForDimension1=[0 0.003 0.3 0.4]  Table=[0 0.45 0.45 0]  ExtrapMethod=Clip  UseLastTableValue=on  InternalRulePriority=Speed  RndMeth=Simplest  InputSameDT=on
  g-lock ECE - 25g/s - 0.45g : Lookup_n-D  NumberOfTableDimensions=1  BreakpointsForDimension1=[0 0.018 0.3 0.4]  Table=[0 0.45 0.45 0]  ExtrapMethod=Clip  UseLastTableValue=on  InternalRulePriority=Speed  RndMeth=Simplest  InputSameDT=on
  g-lock FMVSS  - 16g/s - 0,7g : Lookup_n-D  NumberOfTableDimensions=1  BreakpointsForDimension1=[0 0.04375 0.3 0.4]  Table=[0 0.7 0.7 0]  ExtrapMethod=Clip  UseLastTableValue=on  InternalRulePriority=Speed  RndMeth=Simplest  InputSameDT=on
  g-lock FMVSS - 70g/s - 0.7g : Lookup_n-D  NumberOfTableDimensions=1  BreakpointsForDimension1=[0 0.01 0.3 0.4]  Table=[0 0.7 0.7 0]  ExtrapMethod=Clip  UseLastTableValue=on  InternalRulePriority=Speed  RndMeth=Simplest  InputSameDT=on
  g-lock Vollbremsung - 4g/s - 1g : Lookup_n-D  NumberOfTableDimensions=1  BreakpointsForDimension1=[0 0.25 0.9745 1.2]  Table=[0 1 1 0]  ExtrapMethod=Clip  UseLastTableValue=on  InternalRulePriority=Speed  RndMeth=Simplest  InputSameDT=on
  g_rate : Gain  Gain=5
  pulsetype : Constant  Value=pulsetype
  tilt speed : Gain  Gain=10
  time_const : Constant  Value=-1
  time_const1 : Constant
  zero : Constant  Value=0
  "Pulse_profile " : Outport
  angle in ° : Outport  Port=2
  wires:
  crash angle in rad/1 -> Sin2/1
  tilt speed/1 -> angle in °/1, crash angle in rad/1
  time_const1/1 -> Switch/3
  time_const/1 -> Switch/1
  Switch/1 -> Discrete-Time Integrator4/1
  Discrete-Time Integrator4/1 -> tilt speed/1
  g_rate/1 -> Saturation/1
  Mux1/1 -> Demux/1, g in m/s²/1
  g in m/s²/1 -> "Pulse_profile "/1
  g-lock ECE - 150g/s - 0.45g/1 -> Multiport Switch1/2
  g-lock ECE - 25g/s - 0.45g/1 -> Multiport Switch1/3
  g-lock FMVSS  - 16g/s - 0,7g/1 -> Multiport Switch1/4
  g-lock FMVSS - 70g/s - 0.7g/1 -> Multiport Switch1/5
  "g-lock \" no lock\" - 6g/s - 0.3g"/1 -> Multiport Switch1/6
  "g-lock \" must lock\" - 6g/s - 0.45g"/1 -> Multiport Switch1/7
  g-lock Vollbremsung - 4g/s - 1g/1 -> Multiport Switch1/8
  g-lock Crash - 2000g/s - 30g/1 -> Multiport Switch1/9
  Clock/1 -> Rate Transition/1
  [time] -> g-lock ECE - 150g/s - 0.45g/1
  [time] -> g-lock ECE - 25g/s - 0.45g/1
  [time] -> g-lock FMVSS  - 16g/s - 0,7g/1
  Rate Transition/1 -> [time]
  [time] -> g-lock FMVSS - 70g/s - 0.7g/1
  [time] -> "g-lock \" no lock\" - 6g/s - 0.3g"/1
  [time] -> "g-lock \" must lock\" - 6g/s - 0.45g"/1
  [time] -> g-lock Vollbremsung - 4g/s - 1g/1
  [time] -> g-lock Crash - 2000g/s - 30g/1
  [time] -> Pulse table USNCAP (g)/1
  [time] -> Switch/2
  [time] -> g_rate/1
  [time] -> Puls_Kopfsteinpflaster Meldorf Hindenburgstrasse/1(time in)
  Demux/1 -> Scope/1
  Demux/2 -> Scope/2
  pulsetype/1 -> [pulsetype]
  [pulsetype] -> Multiport Switch1/1
  [pulsetype] -> Multiport Switch2/1
  Puls_Kopfsteinpflaster Meldorf Hindenburgstrasse/1(pulse out [x,y] (g)) -> Demux1/1
  Demux1/1 -> [x_09]
  Demux1/2 -> [y_09]
  zero/1 -> [zero]
  [zero] -> Multiport Switch2/2
  Multiport Switch1/1 -> Mux1/1
  Multiport Switch2/1 -> Mux1/2
  [zero] -> Multiport Switch2/3
  [zero] -> Multiport Switch2/4
  [zero] -> Multiport Switch2/5
  [zero] -> Multiport Switch2/6
  [zero] -> Multiport Switch2/7
  [zero] -> Multiport Switch2/8
  [zero] -> Multiport Switch2/9
  [zero] -> Multiport Switch2/12
  [zero] -> Multiport Switch2/13
  [zero] -> Multiport Switch2/14
  [x_17] -> Multiport Switch1/18
  [x_09] -> Multiport Switch1/10
  Pulse table USNCAP (g)/1 -> Multiport Switch1/11
  [y_09] -> Multiport Switch2/10
  [zero] -> Multiport Switch2/11
  [y_17] -> Multiport Switch2/18
  [zero] -> Multiport Switch2/17
  [zero] -> Multiport Switch2/16
  [zero] -> Multiport Switch2/15
  [y_18] -> Multiport Switch2/19
  [zero] -> Multiport Switch2/20
  [zero] -> Multiport Switch2/21
  [zero] -> Multiport Switch2/22
  [zero] -> Multiport Switch1/22
  [time] -> Pulse table FF27 (g)/1
  Pulse table FF27 (g)/1 -> Multiport Switch1/12
  [time] -> Pulse table ODB40 (g)/1
  [time] -> Pulse table ODB64 (g)/1
  [time] -> Pulse table MPDB (g)/1
  BMW QV72003-3 no-fire lower/1 -> Multiport Switch1/17
  BMW QV72003-3 no-fire upper/1 -> Multiport Switch1/16
  Pulse table MPDB (g)/1 -> Multiport Switch1/15
  Pulse table ODB64 (g)/1 -> Multiport Switch1/14
  Pulse table ODB40 (g)/1 -> Multiport Switch1/13
  Saturation/1 -> Multiport Switch1/21
  Sin2/1 -> Multiport Switch1/20
  [x_18] -> Multiport Switch1/19
  [time] -> BMW QV72003-3 no-fire upper/1
  [time] -> BMW QV72003-3 no-fire lower/1
  Demux2/2 -> [y_17]
  Demux2/1 -> [x_17]
  Puls_GWM_road_C.Morgan/1(pulse out [x,y] (g)) -> Demux2/1
  [time] -> Puls_GWM_road_C.Morgan/1(time in)
  Puls_VW416_Atlas_C.Morgan/1(pulse out [x,y] (g)) -> Demux3/1
  Demux3/1 -> [x_18]
  Demux3/2 -> [y_18]
  [time] -> Puls_VW416_Atlas_C.Morgan/1(time in)

== system eCS_Algo_Simulation/Noisy ==
  Demux : Demux  Tag=STV Demux  Outputs=1
  FromWs : FromWorkspace  Tag=STV FromWs  VariableName=tuvar  SampleTime=0
      SigBuilderData=|
      | common.afterFinalStr = 'Extrapolate'
      | common.sampleTime = 0
      | dataSet.timeRange = [0 0.01]
      | dataSet.name = 'Group 1'
      | sbobj.Groups.Name = 'Group 1'
      | sbobj.Groups.Signals.Name = 'Signal 1'
      | sbobj.Groups.Signals.XData = [0 0.0005 0.001 0.001 0.0015 0.0015 0.002 0.002 0.0025 0.0025 0.003 0.003 0.0035 0.0035 0.004 0.004 0.0045 0.0045 0.005 0.005 0.0055 0.0055 0.006 0.006 0.0065 0.007 0.007 0.0075 0.0075 0.008 0.008 0.0085 0.009 0.0095 0.0095 0.01]
      | sbobj.Groups.Signals.YData = [0 0 1.26 0.79 0.8 0.02 0.02 1.11 1.11 0.8 0.8 0 0 -0.02 1 0.02 0.005 0 0.63 0.65 0.9 0.22 1.09 0.04 0.4 1.58 1.18 1.12 0.32 0.8 0 -0.02 1.12 -0.02 0 0]
      | sbobj.Groups.TimeRange = [0 0.01]
  Signal 1 : Outport  Tag=STV Outport
  wires:
  FromWs/1 -> Demux/1
  Demux/1 -> Signal 1/1

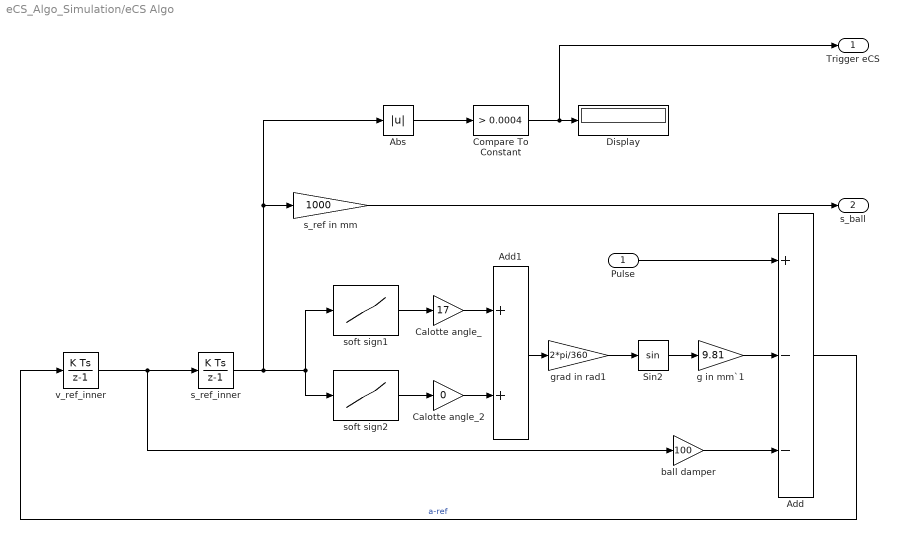
== system eCS_Algo_Simulation/eCS Algo ==
  Pulse : Inport
  Abs : Abs
  Add : Sum  Inputs=+--
  Add1 : Sum
  Calotte angle_ : Gain  Gain=17
  Calotte angle_2 : Gain  Gain=0
  Compare To Constant : simulink/Logic and Bit Operations/Compare To Constant  relop=>  const=0.0004  OutDataTypeStr=uint8
  Display : Display
  Sin2 : Trigonometry
  ball damper : Gain  Gain=100
  g in mm`1 : Gain  Gain=9.81
  grad in rad1 : Gain  Gain=2*pi/360
  s_ref in mm : Gain  Gain=1000
  s_ref_inner : DiscreteIntegrator  SampleTime=-1  LimitOutput=on  UpperSaturationLimit=0.001  LowerSaturationLimit=-0.001  ICPrevOutput=DiscIntNeverNeededParam  ICPrevScaledInput=DiscIntNeverNeededParam
  soft sign1 : Lookup_n-D  NumberOfTableDimensions=1  BreakpointsForDimension1=[-0.002 -0.00002 0.00002 0.002]  Table=[-1 -1 1 1]  ExtrapMethod=Clip  UseLastTableValue=on  InternalRulePriority=Speed  RndMeth=Simplest  InputSameDT=on
  soft sign2 : Lookup_n-D  NumberOfTableDimensions=1  BreakpointsForDimension1="[-0.001 -0.0004 -0.0003 0.0003 0.0004  0.001]"  Table="[-1 -1  0  0 1 1]"  ExtrapMethod=Clip  UseLastTableValue=on  InternalRulePriority=Speed  RndMeth=Simplest  InputSameDT=on
  v_ref_inner : DiscreteIntegrator  SampleTime=-1  ICPrevOutput=DiscIntNeverNeededParam  ICPrevScaledInput=DiscIntNeverNeededParam
  Trigger eCS : Outport
  s_ball : Outport  Port=2
  wires:
  Add/1 -> v_ref_inner/1  "a-ref"
  s_ref in mm/1 -> s_ball/1
  ball damper/1 -> Add/3
  Pulse/1 -> Add/1
  Abs/1 -> Compare To Constant/1
  Sin2/1 -> g in mm`1/1
  Add1/1 -> grad in rad1/1
  Calotte angle_2/1 -> Add1/2
  soft sign2/1 -> Calotte angle_2/1
  Calotte angle_/1 -> Add1/1
  soft sign1/1 -> Calotte angle_/1
  grad in rad1/1 -> Sin2/1
  g in mm`1/1 -> Add/2
  s_ref_inner/1 -> Abs/1, s_ref in mm/1, soft sign2/1, soft sign1/1
  v_ref_inner/1 -> ball damper/1, s_ref_inner/1
  Compare To Constant/1 -> Trigger eCS/1, Display/1

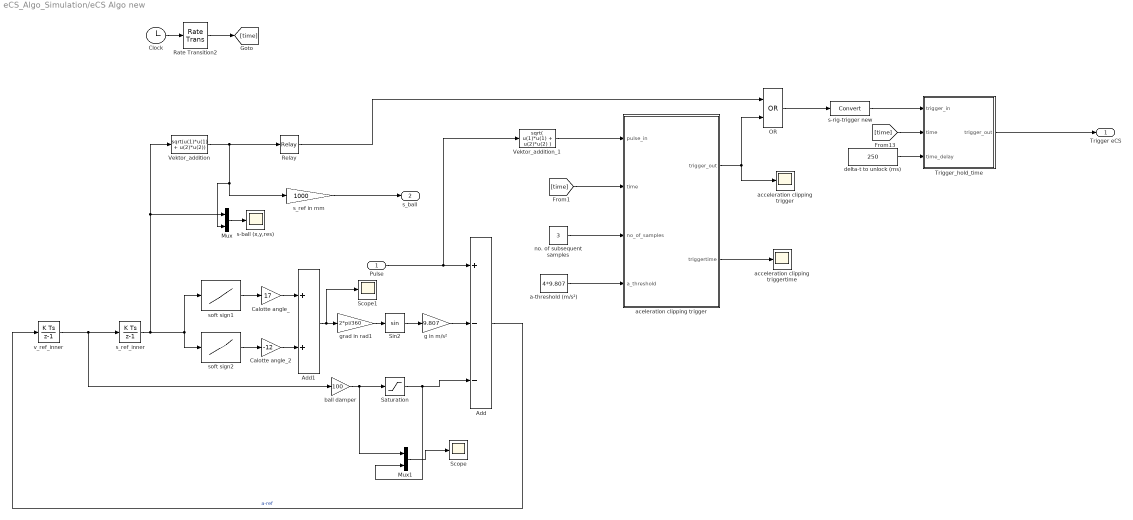
== system eCS_Algo_Simulation/eCS Algo new ==
  Pulse : Inport
  Add : Sum  Inputs=+--
  Add1 : Sum
  Calotte angle_ : Gain  Gain=17
  Calotte angle_2 : Gain  Gain=-12
  Clock : Clock
  Mux : Mux  Inputs=2
  Mux1 : Mux  Inputs=2
  OR : Logic  Operator=OR  AllPortsSameDT=off  OutDataTypeStr=boolean
  Rate Transition2 : RateTransition
  Relay : Relay  OnSwitchValue=0.0004  OffSwitchValue=0.0001
  Saturation : Saturate  UpperLimit=50  LowerLimit=-50
  Scope : Scope
  Scope1 : Scope
  Sin2 : Trigonometry
  Trigger_hold_time : MATLAB Function  TreatAsAtomicUnit=on
  Vektor_addition : Fcn  Expr=sqrt(u(1)*u(1) + u(2)*u(2))
  Vektor_addition_1 : Fcn  Expr=sqrt( u(1)*u(1) + u(2)*u(2) )
  a-threshold (m/s²) : Constant  Value=4*9.807
  acceleration clipping trigger : Scope
  acceleration clipping triggertime : Scope
  aceleration clipping trigger : MATLAB Function  TreatAsAtomicUnit=on
  ball damper : Gain  Gain=100
  delta-t to unlock (ms) : Constant  Value=250  OutMin=[0]
  g in m/s² : Gain  Gain=9.807
  grad in rad1 : Gain  Gain=2*pi/360
  no. of subsequent samples : Constant  Value=3
  s-ball (x,y,res) : Scope
  s-rig-trigger new : DataTypeConversion
  s_ref in mm : Gain  Gain=1000
  s_ref_inner : DiscreteIntegrator  SampleTime=-1  LimitOutput=on  UpperSaturationLimit=0.001  LowerSaturationLimit=-0.001  ICPrevOutput=DiscIntNeverNeededParam  ICPrevScaledInput=DiscIntNeverNeededParam
  soft sign1 : Lookup_n-D  NumberOfTableDimensions=1  BreakpointsForDimension1=[-0.002 -0.00002 0.00002 0.002]  Table=[-1 -1 1 1]  ExtrapMethod=Clip  UseLastTableValue=on  InternalRulePriority=Speed  RndMeth=Simplest  InputSameDT=on
  soft sign2 : Lookup_n-D  NumberOfTableDimensions=1  BreakpointsForDimension1="[-0.001 -0.0005 -0.0004 0.0004 0.0005  0.001]"  Table="[-1 -1  0  0 1 1]"  ExtrapMethod=Clip  UseLastTableValue=on  InternalRulePriority=Speed  RndMeth=Simplest  InputSameDT=on
  v_ref_inner : DiscreteIntegrator  SampleTime=-1  ICPrevOutput=DiscIntNeverNeededParam  ICPrevScaledInput=DiscIntNeverNeededParam
  Trigger eCS : Outport
  s_ball : Outport  Port=2
  wires:
  v_ref_inner/1 -> s_ref_inner/1, ball damper/1
  s_ref_inner/1 -> soft sign1/1, soft sign2/1, Mux/1, Vektor_addition/1
  g in m/s²/1 -> Add/2
  grad in rad1/1 -> Sin2/1
  soft sign1/1 -> Calotte angle_/1
  Calotte angle_/1 -> Add1/1
  soft sign2/1 -> Calotte angle_2/1
  Calotte angle_2/1 -> Add1/2
  Add1/1 -> Scope1/1, grad in rad1/1
  Sin2/1 -> g in m/s²/1
  Vektor_addition/1 -> Relay/1, Mux/2, s_ref in mm/1
  Pulse/1 -> Vektor_addition_1/1, Add/1
  ball damper/1 -> Mux1/1, Saturation/1
  s_ref in mm/1 -> s_ball/1
  Add/1 -> v_ref_inner/1  "a-ref"
  Mux/1 -> s-ball (x,y,res)/1
  Saturation/1 -> Mux1/2, Add/3
  Mux1/1 -> Scope/1
  Clock/1 -> Rate Transition2/1
  aceleration clipping trigger/2(triggertime) -> acceleration clipping triggertime/1
  no. of subsequent samples/1 -> aceleration clipping trigger/3(no_of_samples)
  a-threshold (m/s²)/1 -> aceleration clipping trigger/4(a_threshold)
  aceleration clipping trigger/1(trigger_out) -> acceleration clipping trigger/1, OR/2
  Relay/1 -> OR/1
  Vektor_addition_1/1 -> aceleration clipping trigger/1(pulse_in)
  [time] -> Trigger_hold_time/2(time)
  Rate Transition2/1 -> [time]
  [time] -> aceleration clipping trigger/2(time)
  delta-t to unlock (ms)/1 -> Trigger_hold_time/3(time_delay)
  OR/1 -> s-rig-trigger new/1
  s-rig-trigger new/1 -> Trigger_hold_time/1(trigger_in)
  Trigger_hold_time/1(trigger_out) -> Trigger eCS/1

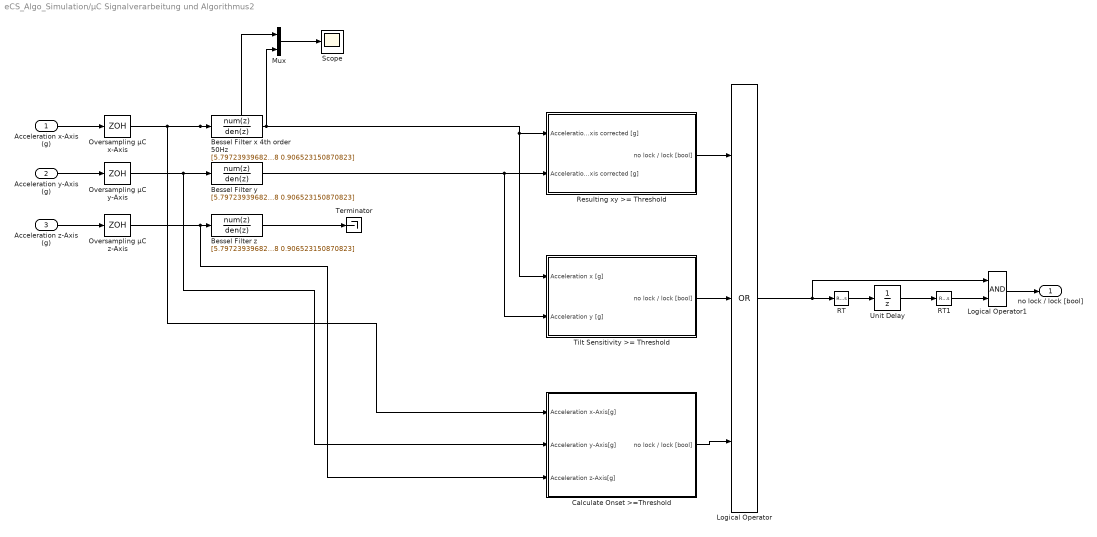
== system eCS_Algo_Simulation/µC Signalverarbeitung und Algorithmus2 ==
  Acceleration x-Axis (g) : Inport
  Acceleration y-Axis (g) : Inport  Port=2
  Acceleration z-Axis (g) : Inport  Port=3
  Bessel Filter x 4th order 50Hz : DiscreteFilter  Numerator=[5.797239396826742e-08 2.318895758730697e-07 3.478343638096045e-07 2.318895758730697e-07 5.797239396826742e-08]  Denominator=[1 -3.902348194587603 5.711314979977801 -3.715489008702718 0.906523150870823]
  Bessel Filter y : DiscreteFilter  Numerator=[5.797239396826742e-08 2.318895758730697e-07 3.478343638096045e-07 2.318895758730697e-07 5.797239396826742e-08]  Denominator=[1 -3.902348194587603 5.711314979977801 -3.715489008702718 0.906523150870823]
  Bessel Filter z : DiscreteFilter  Numerator=[5.797239396826742e-08 2.318895758730697e-07 3.478343638096045e-07 2.318895758730697e-07 5.797239396826742e-08]  Denominator=[1 -3.902348194587603 5.711314979977801 -3.715489008702718 0.906523150870823]
  Calculate Onset >=Threshold : Subsystem
  Logical Operator : Logic  Operator=OR  Inputs=3  AllPortsSameDT=off  OutDataTypeStr=boolean
  Logical Operator1 : Logic  AllPortsSameDT=off  OutDataTypeStr=boolean
  Mux : Mux  Inputs=2
  Oversampling µC x-Axis : ZeroOrderHold  SampleTime=1/10000
  Oversampling µC y-Axis : ZeroOrderHold  SampleTime=1/10000
  Oversampling µC z-Axis : ZeroOrderHold  SampleTime=1/10000
  RT : RateTransition  OutPortSampleTime=0.001
  RT1 : RateTransition  OutPortSampleTime=0.0001
  Resulting xy >= Threshold : Subsystem
  Scope : Scope
  Terminator : Terminator
  Tilt Sensitivity >= Threshold : Subsystem
  Unit Delay : UnitDelay  SampleTime=1/1000
  no lock / lock [bool] : Outport
  wires:
  Acceleration x-Axis (g)/1 -> Oversampling µC x-Axis/1
  Acceleration y-Axis (g)/1 -> Oversampling µC y-Axis/1
  Acceleration z-Axis (g)/1 -> Oversampling µC z-Axis/1
  Resulting xy >= Threshold/1(no lock / lock [bool]) -> Logical Operator/1
  Logical Operator1/1 -> no lock / lock [bool]/1
  Tilt Sensitivity >= Threshold/1(no lock / lock [bool]) -> Logical Operator/2
  Bessel Filter y/1 -> Resulting xy >= Threshold/2(Acceleration y-Axis corrected [g]), Tilt Sensitivity >= Threshold/2(Acceleration y [g])
  Bessel Filter x 4th order 50Hz/1 -> Resulting xy >= Threshold/1(Acceleration x-Axis corrected [g]), Tilt Sensitivity >= Threshold/1(Acceleration x [g]), Mux/2
  Unit Delay/1 -> RT1/1
  Oversampling µC z-Axis/1 -> Bessel Filter z/1, Calculate Onset >=Threshold/3(Acceleration z-Axis[g])
  Calculate Onset >=Threshold/1(no lock / lock [bool]) -> Logical Operator/3
  Oversampling µC y-Axis/1 -> Bessel Filter y/1, Calculate Onset >=Threshold/2(Acceleration y-Axis[g])
  Oversampling µC x-Axis/1 -> Mux/1, Bessel Filter x 4th order 50Hz/1, Calculate Onset >=Threshold/1(Acceleration x-Axis[g])
  Bessel Filter z/1 -> Terminator/1
  Mux/1 -> Scope/1
  Logical Operator/1 -> RT/1, Logical Operator1/1
  RT/1 -> Unit Delay/1
  RT1/1 -> Logical Operator1/2

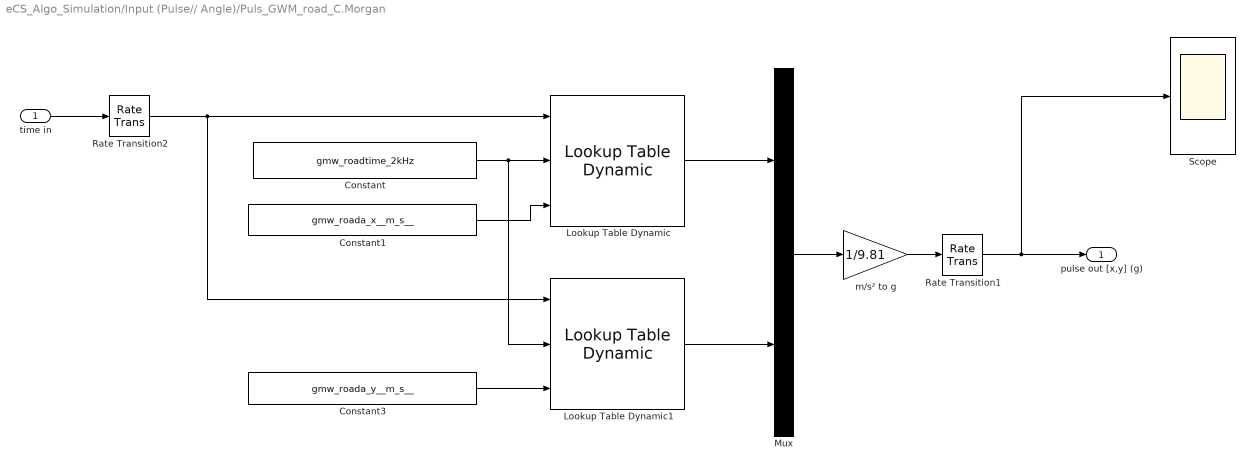
== system eCS_Algo_Simulation/Input (Pulse// Angle)/Puls_GWM_road_C.Morgan ==
  time in : Inport
  Constant : Constant  Value=gmw_roadtime_2kHz
  Constant1 : Constant  Value=gmw_roada_x__m_s__
  Constant3 : Constant  Value=gmw_roada_y__m_s__
  Lookup Table Dynamic : simulink/Lookup Tables/Lookup Table Dynamic  LookUpMeth=Interpolation-Use End Values  OutDataType=fixdt('double')  OutScaling=[]  OutputDataTypeScalingMode=Specify via dialog  OutDataTypeStr=double  DoSatur=off
      settings: SourceProductName=Simulink
  Lookup Table Dynamic1 : simulink/Lookup Tables/Lookup Table Dynamic  LookUpMeth=Interpolation-Use End Values  OutDataType=fixdt('double')  OutScaling=[]  OutputDataTypeScalingMode=Specify via dialog  OutDataTypeStr=double  DoSatur=off
      settings: SourceProductName=Simulink
  Mux : Mux  Inputs=2
  Rate Transition1 : RateTransition
  Rate Transition2 : RateTransition  OutPortSampleTime=1/2000
  Scope : Scope
  m/s² to g : Gain  Gain=1/9.81
  pulse out [x,y] (g) : Outport
  wires:
  Mux/1 -> m/s² to g/1
  m/s² to g/1 -> Rate Transition1/1
  Rate Transition1/1 -> pulse out [x,y] (g)/1, Scope/1
  Constant3/1 -> Lookup Table Dynamic1/3
  Constant/1 -> Lookup Table Dynamic/2, Lookup Table Dynamic1/2
  Constant1/1 -> Lookup Table Dynamic/3
  time in/1 -> Rate Transition2/1
  Lookup Table Dynamic1/1 -> Mux/2
  Rate Transition2/1 -> Lookup Table Dynamic/1, Lookup Table Dynamic1/1
  Lookup Table Dynamic/1 -> Mux/1

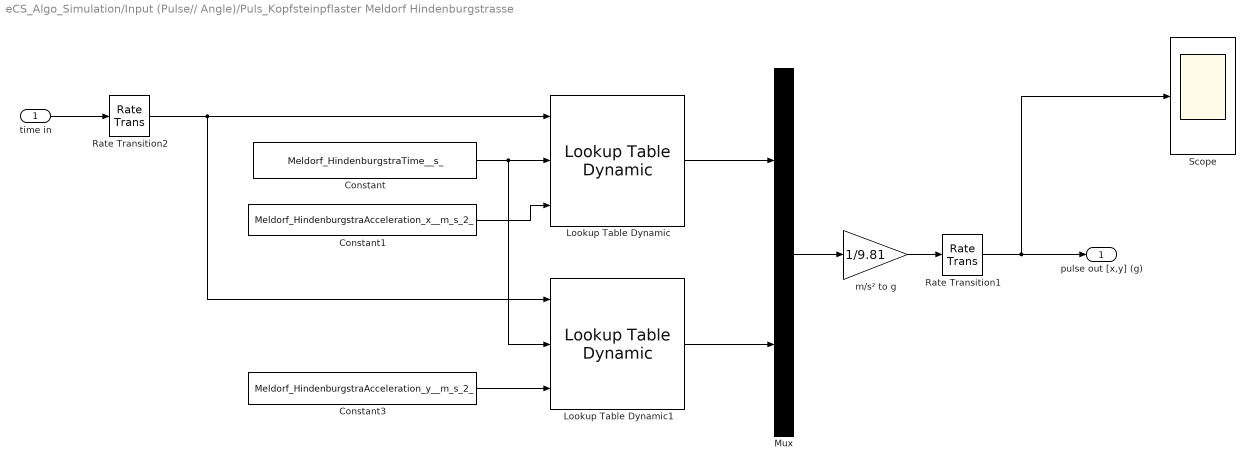
== system eCS_Algo_Simulation/Input (Pulse// Angle)/Puls_Kopfsteinpflaster Meldorf Hindenburgstrasse ==
  time in : Inport
  Constant : Constant  Value=Meldorf_HindenburgstraTime__s_
  Constant1 : Constant  Value=Meldorf_HindenburgstraAcceleration_x__m_s_2_
  Constant3 : Constant  Value=Meldorf_HindenburgstraAcceleration_y__m_s_2_
  Lookup Table Dynamic : simulink/Lookup Tables/Lookup Table Dynamic  LookUpMeth=Interpolation-Use End Values  OutDataType=fixdt('double')  OutScaling=[]  OutputDataTypeScalingMode=Specify via dialog  OutDataTypeStr=double  DoSatur=off
      settings: SourceProductName=Simulink
  Lookup Table Dynamic1 : simulink/Lookup Tables/Lookup Table Dynamic  LookUpMeth=Interpolation-Use End Values  OutDataType=fixdt('double')  OutScaling=[]  OutputDataTypeScalingMode=Specify via dialog  OutDataTypeStr=double  DoSatur=off
      settings: SourceProductName=Simulink
  Mux : Mux  Inputs=2
  Rate Transition1 : RateTransition
  Rate Transition2 : RateTransition  OutPortSampleTime=1/500
  Scope : Scope
  m/s² to g : Gain  Gain=1/9.81
  pulse out [x,y] (g) : Outport
  wires:
  Lookup Table Dynamic/1 -> Mux/1
  Rate Transition2/1 -> Lookup Table Dynamic1/1, Lookup Table Dynamic/1
  Lookup Table Dynamic1/1 -> Mux/2
  time in/1 -> Rate Transition2/1
  Constant1/1 -> Lookup Table Dynamic/3
  Constant/1 -> Lookup Table Dynamic1/2, Lookup Table Dynamic/2
  Constant3/1 -> Lookup Table Dynamic1/3
  Rate Transition1/1 -> Scope/1, pulse out [x,y] (g)/1
  m/s² to g/1 -> Rate Transition1/1
  Mux/1 -> m/s² to g/1

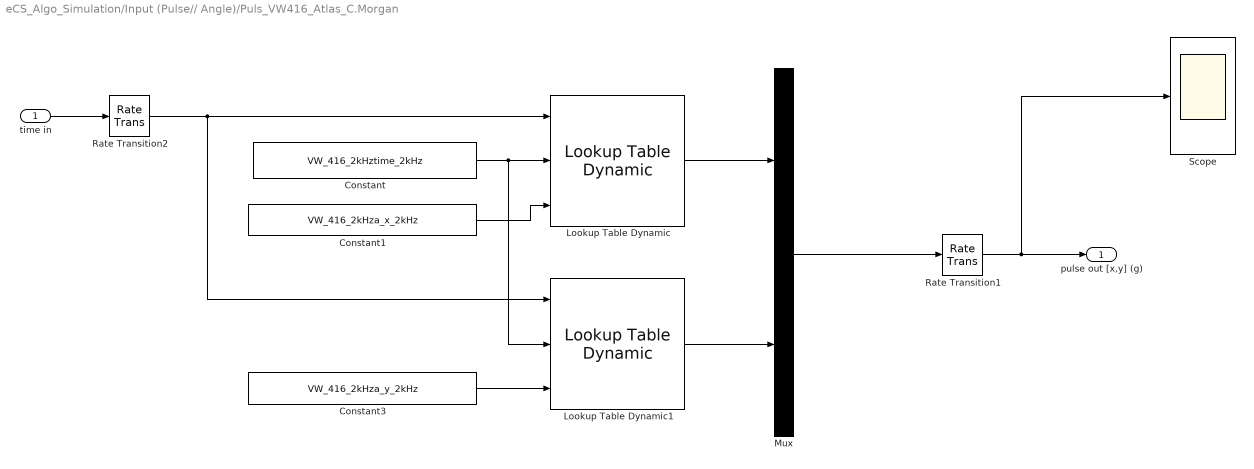
== system eCS_Algo_Simulation/Input (Pulse// Angle)/Puls_VW416_Atlas_C.Morgan ==
  time in : Inport
  Constant : Constant  Value=VW_416_2kHztime_2kHz
  Constant1 : Constant  Value=VW_416_2kHza_x_2kHz
  Constant3 : Constant  Value=VW_416_2kHza_y_2kHz
  Lookup Table Dynamic : simulink/Lookup Tables/Lookup Table Dynamic  LookUpMeth=Interpolation-Use End Values  OutDataType=fixdt('double')  OutScaling=[]  OutputDataTypeScalingMode=Specify via dialog  OutDataTypeStr=double  DoSatur=off
      settings: SourceProductName=Simulink
  Lookup Table Dynamic1 : simulink/Lookup Tables/Lookup Table Dynamic  LookUpMeth=Interpolation-Use End Values  OutDataType=fixdt('double')  OutScaling=[]  OutputDataTypeScalingMode=Specify via dialog  OutDataTypeStr=double  DoSatur=off
      settings: SourceProductName=Simulink
  Mux : Mux  Inputs=2
  Rate Transition1 : RateTransition
  Rate Transition2 : RateTransition  OutPortSampleTime=1/2000
  Scope : Scope
  pulse out [x,y] (g) : Outport
  wires:
  Mux/1 -> Rate Transition1/1
  Rate Transition1/1 -> pulse out [x,y] (g)/1, Scope/1
  Constant3/1 -> Lookup Table Dynamic1/3
  Constant/1 -> Lookup Table Dynamic/2, Lookup Table Dynamic1/2
  Constant1/1 -> Lookup Table Dynamic/3
  time in/1 -> Rate Transition2/1
  Lookup Table Dynamic1/1 -> Mux/2
  Rate Transition2/1 -> Lookup Table Dynamic/1, Lookup Table Dynamic1/1
  Lookup Table Dynamic/1 -> Mux/1
